simulink library "simulink3"  (Simulink 6.0)
settings: Solver=ode45  SolverMode=SingleTasking  StartTime=0.0  StopTime=10.0  RelTol=1e-3
PostLoadFcn:
  | setsysloc(bdroot)
libraries: simulink x33
settings Model: RequirementInfo=9  CovMetricSettings=d  Creator=ricks  LastModifiedBy=andyb  ExtModeAutoUpdateStatusClock=off  ProdHWDeviceType=Microprocessor

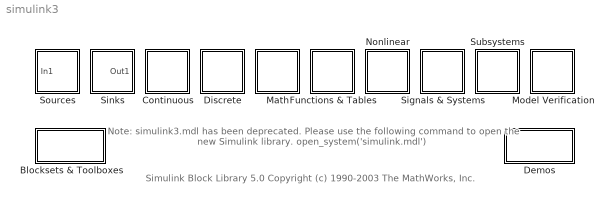
== system simulink3 ==
  note: Simulink Block Library 5.0
      | Copyright (c) 1990-2003 The MathWorks, Inc.
  note: Note: simulink3.mdl has been deprecated.
      | Please use the following command to open the new Simulink library.
      | open_system('simulink.mdl')
  Blocksets & Toolboxes : Subsystem
      settings: OpenFcn=findblib
      mask Display: image(imread('blocksets.bmp','bmp'))
  Continuous : Subsystem
      mask Display: image(imread('continuous.bmp','bmp'))
  Demos : Subsystem
      settings: OpenFcn=demo simulink
      mask Display: image(imread('demos.bmp','bmp'))
  Discrete : Subsystem
      mask Display: image(imread('discrete.bmp','bmp'))
  Functions & Tables : Subsystem
      mask Display: image(imread('functions.bmp','bmp'))
  Math : Subsystem
      mask Display: image(imread('math.bmp','bmp'))
  Model Verification : Subsystem
      mask Display: image(imread('assertion.bmp','bmp'))
  Nonlinear : Subsystem
      mask Display: image(imread('nonlinear.bmp','bmp'))
  Signals & Systems : Subsystem  TreatAsAtomicUnit=on
      mask Display: image(imread('signals.bmp','bmp'))
  Sinks : Subsystem
      mask Display: image(imread('sinks.bmp','bmp'))
  Sources : Subsystem
      mask Display: image(imread('sources.bmp','bmp'))
  Subsystems : Subsystem  TreatAsAtomicUnit=on
      mask Display: image(imread('subsystems.bmp','bmp'))

== system simulink3/Blocksets & Toolboxes ==

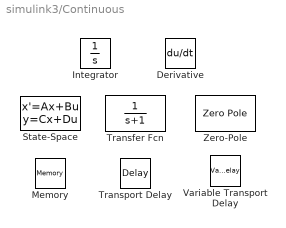
== system simulink3/Continuous ==
  Derivative : Derivative
  Integrator : Integrator
  Memory : Memory
  State-Space : StateSpace
  Transfer Fcn : TransferFcn  Denominator=[1 1]
  Transport Delay : TransportDelay
  Variable Transport Delay : VariableTransportDelay  MaximumDelay=10
  Zero-Pole : ZeroPole  Poles=[0 -1]

== system simulink3/Demos ==

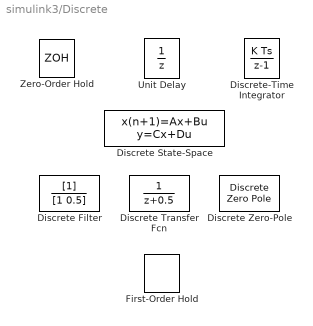
== system simulink3/Discrete ==
  Discrete Transfer Fcn : DiscreteTransferFcn
  Discrete Zero-Pole : DiscreteZeroPole  Poles=[0 0.5]  Gain=1
  Discrete Filter : DiscreteFilter  Denominator=[1 0.5]
  Discrete State-Space : DiscreteStateSpace
  Discrete-Time Integrator : DiscreteIntegrator
  First-Order Hold : simulink/Discrete/First-Order Hold  Ts=1
  Unit Delay : UnitDelay
  Zero-Order Hold : ZeroOrderHold

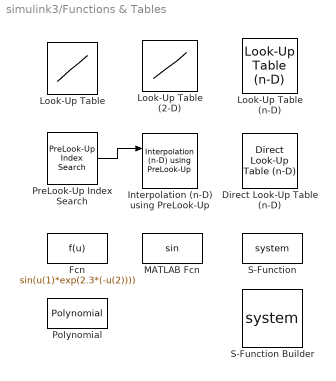
== system simulink3/Functions & Tables ==
  Direct Look-Up Table (n-D) : simulink/Look-Up Tables/Direct Look-Up Table (n-D)  maskTabDims=2  explicitNumDims=1  outDims=Element  tabIsInput=off  mxTable=[4 5 6;16 19 20;10 18 23]  clipFlag=Warning
  Fcn : Fcn  Expr=sin(u(1)*exp(2.3*(-u(2))))
  Interpolation (n-D) using PreLook-Up : simulink/Look-Up Tables/Interpolation (n-D) using PreLook-Up  numDimsPopupSelect=2  explicitNumDims=2  table=sqrt([1:10]'*[1:10])  interpMethod=Linear  extrapMethod=Linear  rangeErrorMode=None
  Look-Up Table : Lookup  InputValues=[-5:5]  OutputValues=tanh([-5:5])  SaturateOnIntegerOverflow=on
  Look-Up Table (2-D) : Lookup2D  RowIndex=[1:3]  ColumnIndex=[1:3]  OutputValues=[4 5 6;16 19 20;10 18 23]  SaturateOnIntegerOverflow=on  InputSameDT=on
  Look-Up Table (n-D) : simulink/Look-Up Tables/Look-Up Table (n-D)  numDimsPopupSelect=2  bp1=[10,22,31]  bp2=[10,22,31]  bp3=[1:3]  bp4=[1:3]  bpcell={ [1:3], [1:3] }  explicitNumDims=2  searchMode=Binary Search  cacheBpFlag=off  vectorInputFlag=off  tableData=[4 5 6;16 19 20;10 18 23]  interpMethod=Linear  extrapMethod=Linear  rangeErrorMode=None
  MATLAB Fcn : MATLABFcn
  Polynomial : simulink/Math Operations/Polynomial  coefs=[ +2.081618890e-019, -1.441693666e-014, +4.719686976e-010, -8.536869453e-006, +1.621573104e-001, -8.087801117e+001 ]
  PreLook-Up Index Search : simulink/Look-Up Tables/PreLook-Up Index Search  bpData=[10:10:100]  searchMode=Binary Search  cacheBpFlag=off  outputFlag=off  extrapMode=Linear Extrapolation  rangeErrorMode=None
  S-Function : S-Function
  S-Function Builder : S-Function  mask(S-Function Builder){}
      mask init:
      | val = [[.9  0.75 0.75 1 1 .9 .9 1]',[1 1 0.75 0.75 .9 .9 1 .9]'];
      | sys = get_param(gcb,'FunctionName');
      settings: CopyFcn=set_param(gcb,'LinkStatus','none')  OpenFcn=sfunctionwizard(gcbh)
      mask Display:
      | plot(val(:,1),val(:,2))
      | disp(sys)
  wires:
  PreLook-Up Index Search/1 -> Interpolation (n-D) using PreLook-Up/1

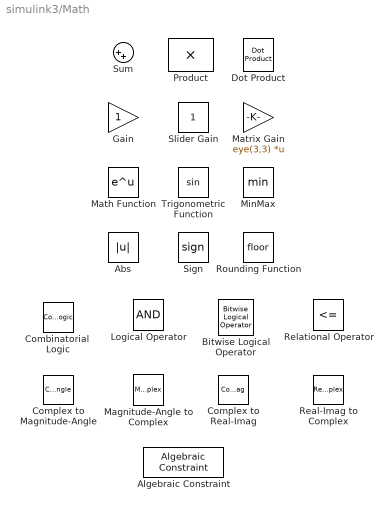
== system simulink3/Math ==
  Abs : Abs  SaturateOnIntegerOverflow=on
  Algebraic Constraint : simulink/Math Operations/Algebraic Constraint  z0=0
  Bitwise Logical Operator : simulink/Logic and Bit Operations/Bitwise Logical Operator  Operator=AND  Operand2='FFFF'
  Combinatorial  Logic : CombinatorialLogic
  Complex to Magnitude-Angle : ComplexToMagnitudeAngle
  Complex to Real-Imag : ComplexToRealImag
  Dot Product : simulink/Math Operations/Dot Product  OutDataType=sfix(16)  OutScaling=2^-10  DoSatur=off
  Gain : Gain  SaturateOnIntegerOverflow=on
  Logical Operator : Logic
  Magnitude-Angle to Complex : MagnitudeAngleToComplex
  Math Function : Math
  Matrix Gain : Gain  Gain=eye(3,3)  Multiplication=Matrix(K*u)  SaturateOnIntegerOverflow=on
  MinMax : MinMax  SaturateOnIntegerOverflow=on  InputSameDT=on
  Product : Product  SaturateOnIntegerOverflow=on  InputSameDT=on
  Real-Imag to Complex : RealImagToComplex
  Relational Operator : RelationalOperator  Operator=<=  InputSameDT=on
  Rounding Function : Rounding
  Sign : Signum
  Slider Gain : simulink/Math Operations/Slider Gain  low=0  gain=1  high=2
  Sum : Sum  Inputs=|++  SaturateOnIntegerOverflow=on  InputSameDT=on
      settings: CopyFcn=set_param(gcbh,'ShowName','off','CopyFcn','')
  Trigonometric Function : Trigonometry

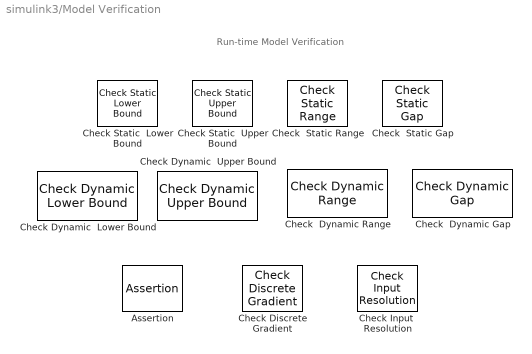
== system simulink3/Model Verification ==
  note: Run-time Model Verification
  Assertion : Assertion
  Check Discrete Gradient : simulink/Model Verification/Check Discrete Gradient  Description=| du / dt | < 1  gradient=1  enabled=on  stopWhenAssertionFail=on  export=off  icon=graphic
  Check  Dynamic Gap : simulink/Model Verification/Check  Dynamic Gap  Description=sig < min || max < sig  enabled=on  stopWhenAssertionFail=on  export=off  icon=graphic
  Check  Dynamic Range : simulink/Model Verification/Check  Dynamic Range  Description=min < sig < max  enabled=on  stopWhenAssertionFail=on  export=off  icon=graphic
  Check  Static Gap : simulink/Model Verification/Check  Static Gap  Description=u <= 0 || 100 <= u  max=100  max_included=on  min=0  min_included=on  enabled=on  stopWhenAssertionFail=on  export=off  icon=graphic
  Check  Static Range : simulink/Model Verification/Check  Static Range  Description=0 <= u <= 100  max=100  max_included=on  min=0  min_included=on  enabled=on  stopWhenAssertionFail=on  export=off  icon=graphic
  Check Dynamic  Lower Bound : simulink/Model Verification/Check Dynamic  Lower Bound  Description=min < sig  Enabled=on  stopWhenAssertionFail=on  export=off  icon=graphic
  Check Dynamic  Upper Bound : simulink/Model Verification/Check Dynamic  Upper Bound  Description=sig < max  enabled=on  stopWhenAssertionFail=on  export=off  icon=graphic
  Check Input  Resolution : simulink/Model Verification/Check Input  Resolution  Description=-Inf < u < +Inf  resolution=1  enabled=on  stopWhenAssertionFail=on  export=off
  Check Static  Lower Bound : simulink/Model Verification/Check Static  Lower Bound  Description=0 <= u  min=0  min_included=on  enabled=on  stopWhenAssertionFail=on  export=off  icon=graphic
  Check Static  Upper Bound : simulink/Model Verification/Check Static  Upper Bound  Description=u <= 0  max=0  max_included=on  enabled=on  stopWhenAssertionFail=on  export=off  icon=graphic

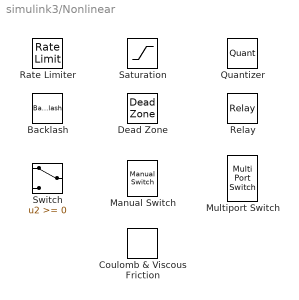
== system simulink3/Nonlinear ==
  Backlash : Backlash
  Coulomb & Viscous Friction : simulink/Discontinuities/Coulomb & Viscous Friction  offset=[1 3 2 0]  gain=1
  Dead Zone : DeadZone  SaturateOnIntegerOverflow=on
  Manual Switch : simulink/Signal Routing/Manual Switch  sw=1  action=0
  Multiport Switch : MultiPortSwitch  Inputs=3  InputSameDT=on
  Quantizer : Quantizer
  Rate Limiter : RateLimiter
  Relay : Relay
  Saturation : Saturate
  Switch : Switch  InputSameDT=on

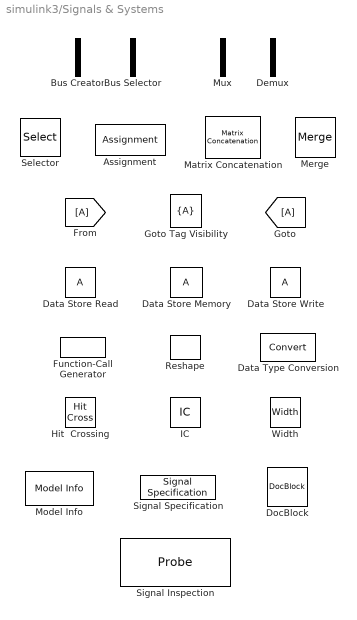
== system simulink3/Signals & Systems ==
  Assignment : Assignment
  Bus Creator : BusCreator  Inputs=2
      settings: CopyFcn=set_param(gcbh,'ShowName','off','CopyFcn','')
  Bus Selector : BusSelector  OutputSignals=signal1,signal2
      settings: CopyFcn=set_param(gcbh,'ShowName','off','CopyFcn','')
  Data Store Memory : DataStoreMemory  DataStoreName=A  InitialValue=0
  Data Store Read : DataStoreRead  DataStoreName=A  SampleTime=0
  Data Store Write : DataStoreWrite  DataStoreName=A  SampleTime=-1
  Data Type Conversion : DataTypeConversion  SaturateOnIntegerOverflow=on  RndMeth=Zero
  Demux : Demux  Outputs=2
      settings: CopyFcn=set_param(gcbh,'ShowName','off','CopyFcn','')
  DocBlock : simulink/Model-Wide Utilities/DocBlock  DocumentType=Text
  Function-Call Generator : simulink/Ports & Subsystems/Function-Call Generator  sample_time=1  numberOfIterations=1
  Goto Tag Visibility : GotoTagVisibility
  Hit  Crossing : HitCross
  IC : InitialCondition
  Matrix Concatenation : simulink/Math Operations/Matrix Concatenation  numInports=2  catMethod=Horizontal
  Merge : Merge
  Model Info : simulink/Model-Wide Utilities/Model Info  InitialBlockCM=none  BlockCM=none  Frame=on  DisplayStringWithTags=Model Info  HorizontalTextAlignment=Center  LeftAlignmentValue=0.5  SourceBlockDiagram=simulink3  TagMaxNumber=20
  Mux : Mux  Inputs=2
      settings: CopyFcn=set_param(gcbh,'ShowName','off','CopyFcn','')
  Reshape : simulink/Math Operations/Reshape  OutputDimensionality=1-D array  OutputDimensions=[1,1]
  Selector : Selector  Elements=[1 3]  InputPortWidth=3
  Signal Inspection : Probe  ProbeSignalDimensions=on
  Signal Specification : SignalSpecification
  Width : Width

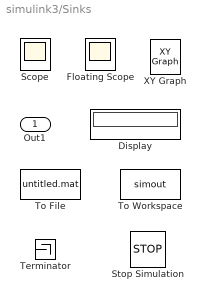
== system simulink3/Sinks ==
  Display : Display
  Floating Scope : Scope
      settings: Floating=on
  Scope : Scope
  Stop Simulation : Stop
  Terminator : Terminator
  To File : ToFile
  To Workspace : ToWorkspace  VariableName=simout  SampleTime=-1  SaveFormat=Structure
  XY Graph : simulink/Sinks/XY Graph  xmin=-1  xmax=1  ymin=-1  ymax=1  st=-1
  Out1 : Outport

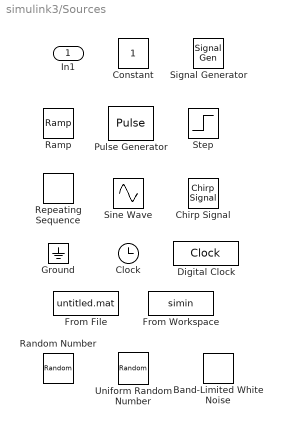
== system simulink3/Sources ==
  In1 : Inport
  Band-Limited White Noise : simulink/Sources/Band-Limited White Noise  Cov=[0.1]  Ts=0.1  seed=[23341]
  Chirp Signal : simulink/Sources/Chirp Signal  f1=0.1  T=100  f2=1
  Clock : Clock
      settings: Decimation=10
  Constant : Constant
  Digital Clock : DigitalClock
  From Workspace : FromWorkspace  VariableName=simin  SampleTime=0
  From File : FromFile  SampleTime=0
  Ground : Ground
  Pulse Generator : DiscretePulseGenerator  PulseType=Time based  PulseWidth=50
  Ramp : simulink/Sources/Ramp  slope=1  start=0  X0=0
  Random Number : RandomNumber  SampleTime=0
  Repeating Sequence : simulink/Sources/Repeating Sequence  rep_seq_t=[0 2]  rep_seq_y=[0 2]
  Signal Generator : SignalGenerator
  Sine Wave : Sin  SampleTime=0
  Step : Step  SampleTime=0
  Uniform Random Number : UniformRandomNumber  SampleTime=0

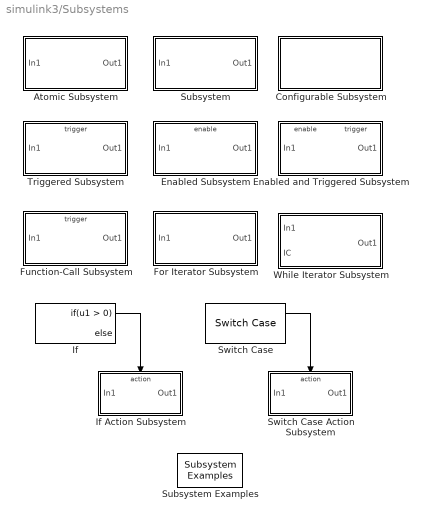
== system simulink3/Subsystems ==
  Atomic Subsystem : Subsystem  TreatAsAtomicUnit=on
      settings: CopyFcn=set_param(gcb,'LinkStatus','none'); set_param(gcb,'Mask','off'); set_param(gcb,'MaskType',''); set_param(gcb,'MaskDescription',''); set_param(gcb,'OpenFcn',''); set_param(gcb,'CopyFcn','')  OpenFcn=open_system(gcb,'force')
      mask Type: Atomic Subsystem
      mask Description: A subsystem block template containing an inport and outport block.
  Configurable Subsystem : Subsystem
      settings: TemplateBlock=master
  Enabled Subsystem : Subsystem  TreatAsAtomicUnit=on
      settings: CopyFcn=set_param(gcb,'LinkStatus','none'); set_param(gcb,'Mask','off'); set_param(gcb,'MaskType',''); set_param(gcb,'MaskDescription',''); set_param(gcb,'OpenFcn',''); set_param(gcb,'CopyFcn','')  OpenFcn=open_system(gcb,'force')
      mask Type: Enabled Subsystem
      mask Description: A subsystem block template containing an enable port, inport and outport block.
  Enabled and Triggered Subsystem : Subsystem  TreatAsAtomicUnit=on
      settings: CopyFcn=set_param(gcb,'LinkStatus','none'); set_param(gcb,'Mask','off'); set_param(gcb,'MaskType',''); set_param(gcb,'MaskDescription',''); set_param(gcb,'OpenFcn',''); set_param(gcb,'CopyFcn','')  OpenFcn=open_system(gcb,'force')
      mask Type: Enabled And Triggered Subsystem
      mask Description: A subsystem block template containing an enable port, trigger port, inport and outport block.
  For Iterator Subsystem : Subsystem  TreatAsAtomicUnit=on
      settings: CopyFcn=set_param(gcb,'LinkStatus','none'); set_param(gcb,'Mask','off'); set_param(gcb,'MaskType',''); set_param(gcb,'MaskDescription',''); set_param(gcb,'OpenFcn',''); set_param(gcb,'CopyFcn','')  OpenFcn=open_system(gcb,'force')
      mask Type: For Iterator Subsystem
      mask Description: A subsystem block template containing a for iterator, inport and outport block.
  Function-Call Subsystem : Subsystem  TreatAsAtomicUnit=on
      settings: CopyFcn=set_param(gcb,'LinkStatus','none'); set_param(gcb,'Mask','off'); set_param(gcb,'MaskType',''); set_param(gcb,'MaskDescription',''); set_param(gcb,'OpenFcn',''); set_param(gcb,'CopyFcn','')  OpenFcn=open_system(gcb,'force')
      mask Type: Function-Call Subsystem
      mask Description: A subsystem block template containing a function-call trigger port, inport and outport block.
  If : If
  If Action Subsystem : Subsystem  TreatAsAtomicUnit=on
      settings: CopyFcn=set_param(gcb,'LinkStatus','none'); set_param(gcb,'Mask','off'); set_param(gcb,'MaskType',''); set_param(gcb,'MaskDescription',''); set_param(gcb,'OpenFcn',''); set_param(gcb,'CopyFcn','')  OpenFcn=open_system(gcb,'force')
      mask Type: If Action Subsystem
      mask Description: A subsystem block template containing an action port, inport and outport block.
  Subsystem : Subsystem
      settings: CopyFcn=set_param(gcb,'LinkStatus','none'); set_param(gcb,'Mask','off'); set_param(gcb,'MaskType',''); set_param(gcb,'MaskDescription',''); set_param(gcb,'OpenFcn',''); set_param(gcb,'CopyFcn','')  OpenFcn=open_system(gcb,'force')
      mask Type: Virtual Subsystem
      mask Description: A subsystem block template containing an inport and outport block.
  Subsystem Examples : simulink/Ports & Subsystems/Subsystem Examples
  Switch Case : SwitchCase
  Switch Case Action Subsystem : Subsystem  TreatAsAtomicUnit=on
      settings: CopyFcn=set_param(gcb,'LinkStatus','none'); set_param(gcb,'Mask','off'); set_param(gcb,'MaskType',''); set_param(gcb,'MaskDescription',''); set_param(gcb,'OpenFcn',''); set_param(gcb,'CopyFcn','')  OpenFcn=open_system(gcb,'force')
      mask Type: Switch Case Action Subsystem
      mask Description: A subsystem block template containing an action port, inport and outport block.
  Triggered Subsystem : Subsystem  TreatAsAtomicUnit=on
      settings: CopyFcn=set_param(gcb,'LinkStatus','none'); set_param(gcb,'Mask','off'); set_param(gcb,'MaskType',''); set_param(gcb,'MaskDescription',''); set_param(gcb,'OpenFcn',''); set_param(gcb,'CopyFcn','')  OpenFcn=open_system(gcb,'force')
      mask Type: Triggered Subsystem
      mask Description: A subsystem block template containing a trigger port, inport and outport block.
  While Iterator Subsystem : Subsystem  TreatAsAtomicUnit=on
      settings: CopyFcn=set_param(gcb,'LinkStatus','none'); set_param(gcb,'Mask','off'); set_param(gcb,'MaskType',''); set_param(gcb,'MaskDescription',''); set_param(gcb,'OpenFcn',''); set_param(gcb,'CopyFcn','')  OpenFcn=open_system(gcb,'force')
      mask Type: While Iterator Subsystem
      mask Description: A subsystem block template containing a while iterator, inport and outport block.
  wires:
  If/1 -> If Action Subsystem/Action
  Switch Case/1 -> Switch Case Action Subsystem/Action

== system simulink3/Subsystems/Atomic Subsystem ==
  In1 : Inport
  Out1 : Outport
  wires:
  In1/1 -> Out1/1

== system simulink3/Subsystems/Configurable Subsystem ==

== system simulink3/Subsystems/Enabled Subsystem ==
  In1 : Inport
  Enable : EnablePort
  Out1 : Outport
  wires:
  In1/1 -> Out1/1

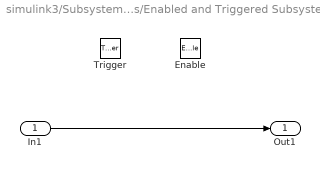
== system simulink3/Subsystems/Enabled and Triggered Subsystem ==
  In1 : Inport
  Enable : EnablePort
  Trigger : TriggerPort
  Out1 : Outport
  wires:
  In1/1 -> Out1/1

== system simulink3/Subsystems/For Iterator Subsystem ==
  In1 : Inport
  For Iterator : ForIterator
  Out1 : Outport
  wires:
  In1/1 -> Out1/1

== system simulink3/Subsystems/Function-Call Subsystem ==
  In1 : Inport
  function : TriggerPort  TriggerType=function-call
  Out1 : Outport
  wires:
  In1/1 -> Out1/1

== system simulink3/Subsystems/If Action Subsystem ==
  In1 : Inport
  Action Port : ActionPort  ActionType=then
  Out1 : Outport
  wires:
  In1/1 -> Out1/1

== system simulink3/Subsystems/Subsystem ==
  In1 : Inport
  Out1 : Outport
  wires:
  In1/1 -> Out1/1

== system simulink3/Subsystems/Switch Case Action Subsystem ==
  In1 : Inport
  Action Port : ActionPort  ActionType=case
  Out1 : Outport
  wires:
  In1/1 -> Out1/1

== system simulink3/Subsystems/Triggered Subsystem ==
  In1 : Inport
  Trigger : TriggerPort
  Out1 : Outport
  wires:
  In1/1 -> Out1/1

== system simulink3/Subsystems/While Iterator Subsystem ==
  In1 : Inport
  IC : Inport  Port=2
  While Iterator : WhileIterator
  Out1 : Outport
  wires:
  In1/1 -> Out1/1
  IC/1 -> While Iterator/2
